simulink model "topmain"  (R2020b)
settings: configuration reference "configurationSettings" (kept outside this file)
settings Model: DataDictionary=topmain.sldd  Creator=ravenst1  LastModifiedBy=ravenst1
settings ConfigSetRef: SourceName=configurationSettings

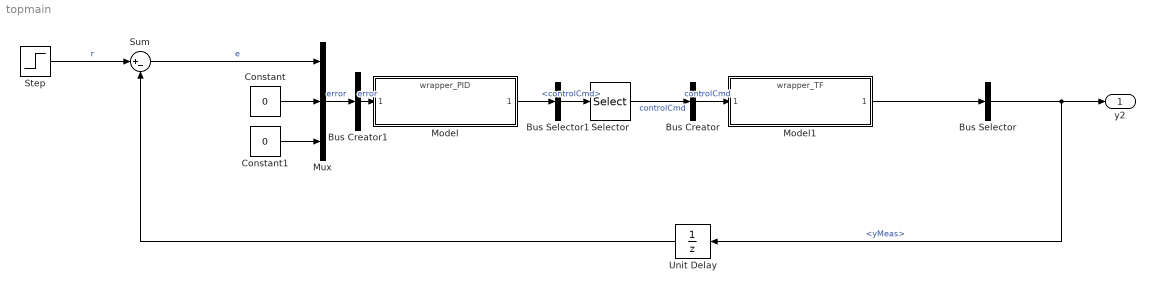
== system topmain ==
  Bus Creator : BusCreator  Inputs=1
  Bus Creator1 : BusCreator  Inputs=1  OutDataTypeStr=Bus: pcssp_PID_inBus
  Bus Selector : BusSelector  OutputSignals=yMeas
  Bus Selector1 : BusSelector  OutputSignals=controlCmd
  Constant : Constant  Value=0
  Constant1 : Constant  Value=0
  Model : ModelReference  ModelNameDialog=wrapper_PID.slx  SimulationMode=Normal  ModelReferenceVersion=1.8
  Model1 : ModelReference  ModelNameDialog=wrapper_TF.slx  SimulationMode=Normal  ModelReferenceVersion=1.5
  Mux : Mux  Inputs=3
  Selector : Selector  InputPortWidth=3  IndexOptions=Index vector (dialog)  Indices=1  OutputSizes=1
  Step : Step  Time=2  SampleTime=0
  Sum : Sum  Inputs=|+-
  Unit Delay : UnitDelay  SampleTime=-1  HasFrameUpgradeWarning=on
  y2 : Outport
  wires:
  Bus Creator/1 -> Model1/1  "controlCmd"
  Sum/1 -> Mux/1  "e"
  Bus Selector/1 -> Unit Delay/1, y2/1  "<yMeas>"
  Mux/1 -> Bus Creator1/1  "error"
  Constant/1 -> Mux/2
  Bus Selector1/1 -> Selector/1  "<controlCmd>"
  Selector/1 -> Bus Creator/1  "controlCmd"
  Model/1 -> Bus Selector1/1
  Constant1/1 -> Mux/3
  Unit Delay/1 -> Sum/2
  Step/1 -> Sum/1  "r"
  Model1/1 -> Bus Selector/1
  Bus Creator1/1 -> Model/1  "error"
